simulink model "CoTemp"  (R2016b)
settings: configuration reference "CodeGenConfigSet" (kept outside this file)
values from neighbouring files (symbols this model uses):
  CoTemp_rClgDes_C = Calibration.Parameter    [init_CoTemp.m]
  CoTemp_tEngDes_C = Calibration.Parameter    [init_CoTemp.m]
settings Model: Creator=lenovo  LastModifiedBy=lenovo
settings ConfigSetRef: SourceLocation=Base Workspace

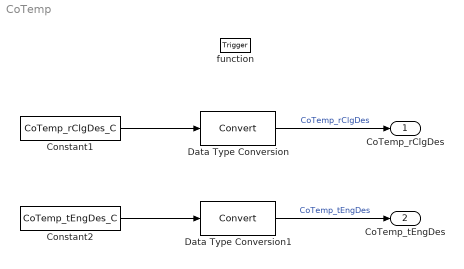
== system CoTemp ==
  function : TriggerPort  TriggerType=function-call  VariantControl=Variant
  Constant1 : Constant  Value=CoTemp_rClgDes_C
  Constant2 : Constant  Value=CoTemp_tEngDes_C
  Data Type Conversion : DataTypeConversion
  Data Type Conversion1 : DataTypeConversion
  CoTemp_rClgDes : Outport  Tag=%  Description=Cooling requirement of the combustion engine  OutMin=-300  OutMax=300  OutDataTypeStr=Prc_100_rate
  CoTemp_tEngDes : Outport  Tag=deg  Description=Coolant temperature of combustion engine  Port=2  OutMin=-3549  OutMax=3003  OutDataTypeStr=Temp_deg
  wires:
  Constant1/1 -> Data Type Conversion/1
  Constant2/1 -> Data Type Conversion1/1
  Data Type Conversion/1 -> CoTemp_rClgDes/1  "CoTemp_rClgDes"
  Data Type Conversion1/1 -> CoTemp_tEngDes/1  "CoTemp_tEngDes"
